simulink model "vspriklad1_sim"  (R2018b)
settings: Solver=VariableStepAuto  StartTime=0.0  StopTime=time  RelTol=1e-3
undefined symbols (not defined in the file): D, I, k1, k2, P, r, rpid
settings Model: Creator=Evka  LastModifiedBy=Evka

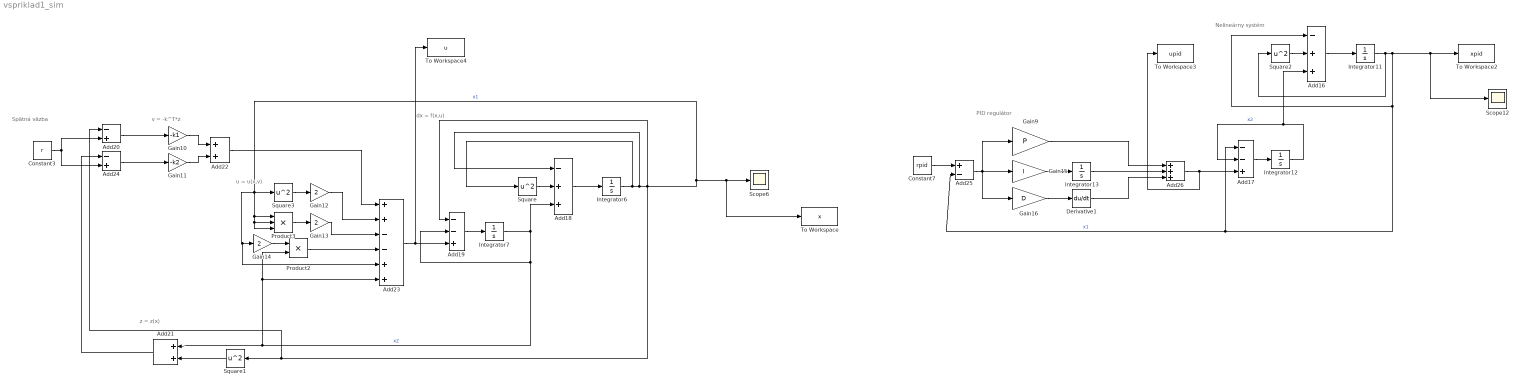
== system vspriklad1_sim ==
  note: Nelineárny systém
  note: PID regulátor
  note: u = u(x,v)
  note: Spätná väzba
  note: z = z(x)
  note: dx = f(x,u)
  note: v = -k^T*z
  Add16 : Sum  Inputs=-++
  Add17 : Sum  Inputs=--+
  Add18 : Sum  Inputs=-++
  Add19 : Sum  Inputs=--+
  Add20 : Sum  Inputs=-+
  Add21 : Sum
  Add22 : Sum
  Add23 : Sum  Inputs=++--++
  Add24 : Sum  Inputs=-+
  Add25 : Sum  Inputs=+-
  Add26 : Sum  Inputs=+++
  Constant3 : Constant  Value=r
  Constant7 : Constant  Value=rpid
  Derivative1 : Derivative
  Gain10 : Gain  Gain=-k1
  Gain11 : Gain  Gain=-k2
  Gain12 : Gain  Gain=2
  Gain13 : Gain  Gain=2
  Gain14 : Gain  Gain=2
  Gain15 : Gain  Gain=I
  Gain16 : Gain  Gain=D
  Gain9 : Gain  Gain=P
  Integrator{6..7,11..13} (5 alike) : Integrator
  Product2 : Product
  Product3 : Product  Inputs=3
  Scope12 : Scope
  Scope6 : Scope
  Square{,1..3} (4 alike) : Math  Operator=square  SaturateOnIntegerOverflow=on
  To Workspace : ToWorkspace  VariableName=x  SaveFormat=Timeseries  SampleTime=-1
  To Workspace2 : ToWorkspace  VariableName=xpid  SaveFormat=Timeseries  SampleTime=-1
  To Workspace3 : ToWorkspace  VariableName=upid  SaveFormat=Timeseries  SampleTime=-1
  To Workspace4 : ToWorkspace  VariableName=u  SaveFormat=Timeseries  SampleTime=-1
  wires:
  Constant7/1 -> Add25/1
  Derivative1/1 -> Add26/3
  Add26/1 -> To Workspace3/1, Add17/3
  Square2/1 -> Add16/2
  Gain16/1 -> Derivative1/1
  Integrator12/1 -> Add16/3, Add17/2  "x2"
  Gain9/1 -> Add26/1
  Integrator13/1 -> Add26/2
  Gain15/1 -> Integrator13/1
  Add25/1 -> Gain16/1, Gain15/1, Gain9/1
  Add16/1 -> Integrator11/1
  Integrator11/1 -> Square2/1, Scope12/1, To Workspace2/1, Add16/1, Add17/1, Add25/2  "x1"
  Add17/1 -> Integrator12/1
  Product3/1 -> Gain13/1
  Square/1 -> Add18/2
  Gain12/1 -> Add23/2
  Add23/1 -> To Workspace4/1, Add19/3
  Add20/1 -> Gain10/1
  Product2/1 -> Add23/4
  Integrator6/1 -> To Workspace/1, Scope6/1, Product3/3, Product3/2, Product3/1, Square3/1, Add23/5, Gain14/1, Add20/1, Square1/1, Add19/1, Add18/1, Square/1  "x1"
  Square3/1 -> Gain12/1
  Add18/1 -> Integrator6/1
  Constant3/1 -> Add20/2, Add24/2
  Add21/1 -> Add24/1
  Add24/1 -> Gain11/1
  Gain11/1 -> Add22/2
  Gain14/1 -> Product2/1
  Square1/1 -> Add21/2
  Integrator7/1 -> Add21/1, Product2/2, Add23/6, Add19/2, Add18/3  "x2"
  Add22/1 -> Add23/1
  Gain10/1 -> Add22/1
  Add19/1 -> Integrator7/1
  Gain13/1 -> Add23/3
